simulink model "scheme2_2"  (R2021a)
settings: Solver=ode1  StartTime=0.0  StopTime=45  FixedStep=Tp  RelTol=1e-3
values from neighbouring files (symbols this model uses):
  k = 6    [exercise1.m]    (also in exercise2.m)
  kp = 1.6    [exercise1.m]    (also in exercise2.m)
  T_1 = 5.9    [exercise1.m]    (also in exercise2.m)
  T_2 = 0.8    [exercise1.m]    (also in exercise2.m)
  Td = 0.08    [exercise1.m]    (also in exercise2.m)
  Ti = 6    [exercise1.m]    (also in exercise2.m)
  Tp = 0.01    [exercise1.m]    (also in exercise2.m)
undefined symbols (not defined in the file or in its folder): magnitude
settings Model: Creator=AgraWoodAdmin  LastModifiedBy=AgraWoodAdmin

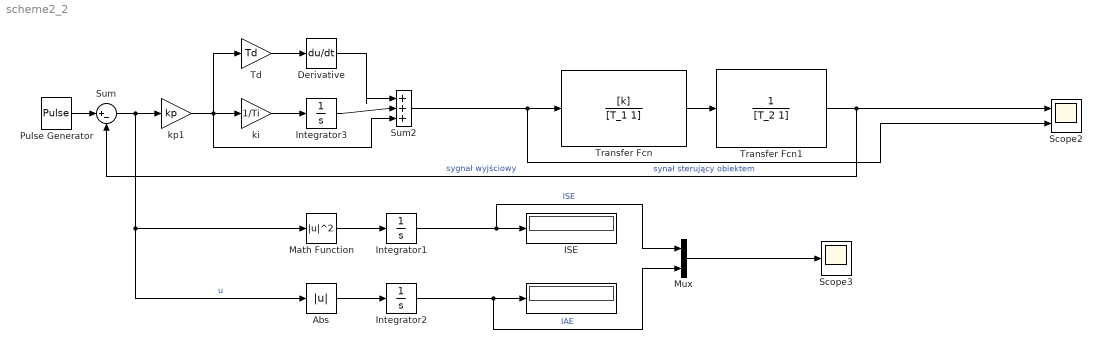
== system scheme2_2 ==
  " " : Display
  Abs : Abs  SaturateOnIntegerOverflow=on
  Derivative : Derivative
  ISE : Display
  Integrator1 : Integrator  InitialCondition=Tp
  Integrator2 : Integrator
  Integrator3 : Integrator
  Math Function : Math  Operator=magnitude^2  SignedPower=on  SaturateOnIntegerOverflow=on
  Mux : Mux  Inputs=2
  Pulse Generator : DiscretePulseGenerator  PulseType=Time based  Period=45  PulseWidth=50
  Scope2 : Scope  NumInputPorts=2
  Scope3 : Scope
  Sum : Sum  Inputs=|+-
  Sum2 : Sum  Inputs=|+++  SaturateOnIntegerOverflow=on
  Td : Gain  Gain=Td  SaturateOnIntegerOverflow=on  OutDataTypeStr=Inherit: Same as input  ParamDataTypeStr=Inherit: Same as input
  Transfer Fcn : TransferFcn  Numerator=[k]  Denominator=[T_1 1]
  Transfer Fcn1 : TransferFcn  Denominator=[T_2 1]
  ki : Gain  Gain=1/Ti  SaturateOnIntegerOverflow=on  OutDataTypeStr=Inherit: Same as input  ParamDataTypeStr=Inherit: Same as input
  kp1 : Gain  Gain=kp  SaturateOnIntegerOverflow=on  OutDataTypeStr=Inherit: Same as input  ParamDataTypeStr=Inherit: Same as input
  wires:
  Pulse Generator/1 -> Sum/1
  Integrator1/1 -> Mux/1, ISE/1  "ISE"
  Derivative/1 -> Sum2/1
  Td/1 -> Derivative/1
  Sum2/1 -> Scope2/2, Transfer Fcn/1  "synał sterujący obiektem"
  Math Function/1 -> Integrator1/1
  ki/1 -> Integrator3/1
  Integrator2/1 -> Mux/2, " "/1  "IAE"
  kp1/1 -> Td/1, Sum2/3, ki/1
  Abs/1 -> Integrator2/1
  Integrator3/1 -> Sum2/2
  Sum/1 -> kp1/1, Math Function/1, Abs/1  "u"
  Mux/1 -> Scope3/1
  Transfer Fcn/1 -> Transfer Fcn1/1
  Transfer Fcn1/1 -> Scope2/1, Sum/2  "sygnał wyjściowy"
